simulink model "RCAC_ESC_KF_SISO_line_change"  (R2023a)
settings: Solver=FixedStepDiscrete  StartTime=0.0  StopTime=k_end  FixedStep=1  RelTol=1e-3
values from neighbouring files (symbols this model uses):
  ref_val = 5    [run_RCAC_ESC_KF_SISO_line_change.m]
  u_init = 0    [run_RCAC_ESC_KF_SISO_line_change.m]
settings Model: Creator=Juan Augusto Paredes  LastModifiedBy=Juan Augusto Paredes

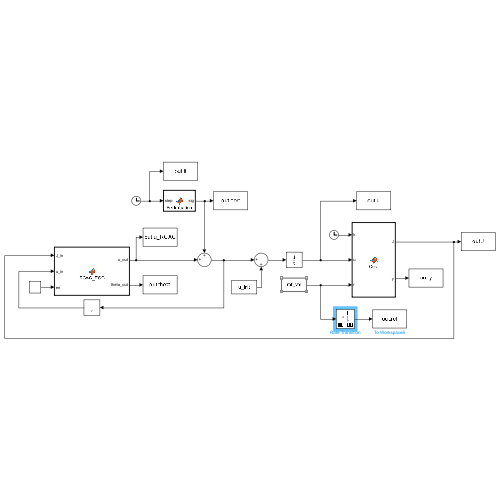
[thumbnail: Simulink's stored preview of the top-level diagram]
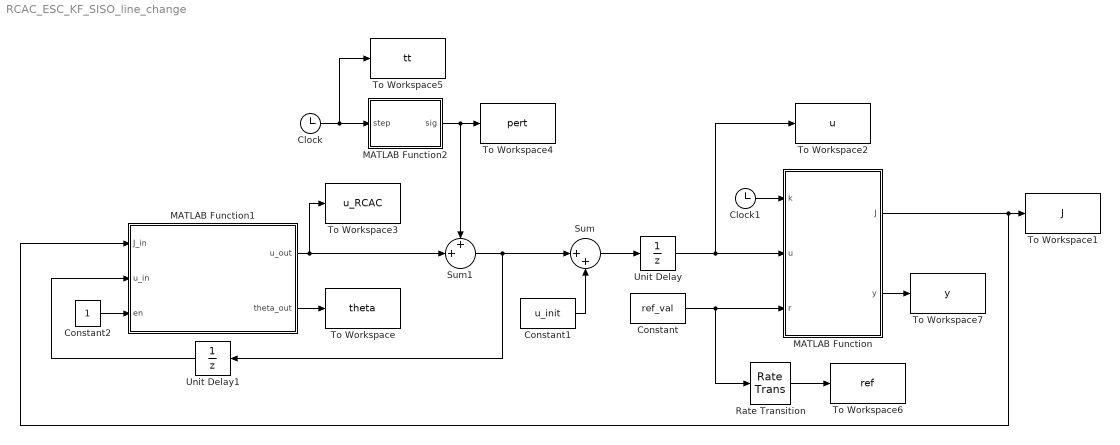
== system RCAC_ESC_KF_SISO_line_change ==
  Clock : Clock
  Clock1 : Clock
  Constant : Constant  Value=ref_val
  Constant1 : Constant  Value=u_init
  Constant2 : Constant
  MATLAB Function : MATLAB Function  TreatAsAtomicUnit=on
  MATLAB Function1 : MATLAB Function  TreatAsAtomicUnit=on
  MATLAB Function2 : MATLAB Function  TreatAsAtomicUnit=on
  Rate Transition : RateTransition  OutPortSampleTime=1
  Sum : Sum  Inputs=|++
  Sum1 : Sum  Inputs=++|
  To Workspace : ToWorkspace  VariableName=theta  SampleTime=-1
  To Workspace1 : ToWorkspace  VariableName=J  SampleTime=-1
  To Workspace2 : ToWorkspace  VariableName=u  SampleTime=-1
  To Workspace3 : ToWorkspace  VariableName=u_RCAC  SampleTime=-1
  To Workspace4 : ToWorkspace  VariableName=pert  SampleTime=-1
  To Workspace5 : ToWorkspace  VariableName=tt  SampleTime=-1
  To Workspace6 : ToWorkspace  VariableName=ref  SampleTime=-1
  To Workspace7 : ToWorkspace  VariableName=y  SampleTime=-1
  Unit Delay : UnitDelay  InitialCondition=u_init  SampleTime=-1  HasFrameUpgradeWarning=on
  Unit Delay1 : UnitDelay  SampleTime=-1  HasFrameUpgradeWarning=on
  wires:
  Unit Delay/1 -> To Workspace2/1, MATLAB Function/2(u)
  Sum/1 -> Unit Delay/1
  MATLAB Function1/1(u_out) -> To Workspace3/1, Sum1/2
  MATLAB Function2/1(sig) -> Sum1/1, To Workspace4/1
  Clock/1 -> To Workspace5/1, MATLAB Function2/1(step)
  Unit Delay1/1 -> MATLAB Function1/2(u_in)
  MATLAB Function/1(J) -> MATLAB Function1/1(J_in), To Workspace1/1
  MATLAB Function1/2(theta_out) -> To Workspace/1
  Constant2/1 -> MATLAB Function1/3(en)
  Sum1/1 -> Unit Delay1/1, Sum/1
  Constant1/1 -> Sum/2
  Constant/1 -> MATLAB Function/3(r), Rate Transition/1
  Clock1/1 -> MATLAB Function/1(k)
  MATLAB Function/2(y) -> To Workspace7/1
  Rate Transition/1 -> To Workspace6/1

== matlab function RCAC_ESC_KF_SISO_line_change/MATLAB Function1 ==
  settings: updateMethod=DISCRETE  sampleTime=1
  data: J_in input size=1; u_out output size=1; u_in input size=1; en input size=1; theta_out output size=20; Nc parameter size=1
function [u_out, theta_out] = RCAC_ESC(J_in, u_in, en, Nc)

persistent Grad_Est DDRCAC_Cont uouttemp thetaouttemp opts

if isempty(uouttemp)
    opts = RCAC_ESC_KF_SISO_line_change_define_opts();
    Grad_Est = grad_est_KF(opts.lu, opts.lz, opts.indi, opts.P0_G, opts.Q, opts.R);
    DDRCAC_Cont = DDRCAC(opts.lu, opts.lz, opts.Nc, opts.P0_C, opts.Ru, opts.nu);
    uouttemp = 0.0;
    thetaouttemp = zeros(2*Nc,1); 
end

theta_out = zeros(20,1); %Due to Max number for Nc = 10, can adjust by changing theta_out size

if en > 0.5
    %% Gradient estimation
    [Grad_Est, grad] = Grad_Est.oneStep(u_in, J_in, en);
    
    %% Gradient to Nf (SISO)
    gradNorm = abs(grad);
    gradNorm(gradNorm<=opts.epsi) = opts.epsi;
    Nf = grad./gradNorm;
    
    %% RCAC with Nf (DDRCAC)
    [DDRCAC_Cont, uouttemp, thetaouttemp] = DDRCAC_Cont.oneStep(u_in, J_in, Nf, 0);

end

u_out = uouttemp(1,1);
theta_out(1:2*Nc,1) = thetaouttemp(1:2*Nc,1);

end

== matlab function RCAC_ESC_KF_SISO_line_change/MATLAB Function ==
  settings: updateMethod=DISCRETE
  data: k input size=1; u input size=1; J output size=1; r input size=1; k_jump parameter size=1; y output size=1
function [J,y] = Cost(k,u,r,k_jump)

    [J,y] = CostFcnSISO_line_change(k,k_jump,u,r);

end

== matlab function RCAC_ESC_KF_SISO_line_change/MATLAB Function2 ==
  settings: updateMethod=DISCRETE
  data: step input size=1; sig output size=1
function sig = Perturbation(step)
    sig = PertFcnSISO(step);
end
